simulink model "DC_Motor_speed_current_ctrl"  (R2021b)
settings: Solver=FixedStepAuto  StartTime=0.0  StopTime=2  FixedStep=5e-6  RelTol=1e-3
values from neighbouring files (symbols this model uses):
  B = 6.03e-6    (= 6.03e-06)    [DCMachine_cal.m]    (also in DC_Motor_speed_current_ctrl_cal.m = 0)
  I_rated = 74    [DC_Motor_speed_current_ctrl_cal.m]
  J = 1.06e-6    (= 1.06e-06)    [DCMachine_cal.m]    (also in DC_Motor_speed_current_ctrl_cal.m = 0.156)
  Kc = La/Td    (= 2.93)    [DC_Motor_speed_current_ctrl_cal.m]
  Kn = (J*K2)/(K1*Kphi*2*delta)    (= 65.9693860709)    [DC_Motor_speed_current_ctrl_cal.m]
  Kphi = 1.41e-2    (= 0.0141)    [DCMachine_cal.m]    (also in DC_Motor_speed_current_ctrl_cal.m = 1.18236661951)
  La = 120e-3    (= 0.12)    [DCMachine_cal.m]    (also in DC_Motor_speed_current_ctrl_cal.m = 0.00293)
  m_L = 0    [DC_Motor_speed_current_ctrl_cal.m]
  Ra = 7    [DCMachine_cal.m]    (also in DC_Motor_speed_current_ctrl_cal.m = 0.18)
  Tc = Ta    (= 0.0162777777778)    [DC_Motor_speed_current_ctrl_cal.m]
  Tn = 4*delta    (= 0.004)    [DC_Motor_speed_current_ctrl_cal.m]
  Vt = 6    [DCMachine_cal.m]    (also in DC_Motor_speed_current_ctrl_cal.m = 230)
  w_rpm = 1750    [DC_Motor_speed_current_ctrl_cal.m]
settings Model: Creator=jmvir  LastModifiedBy=Dinh-Tuyen Le

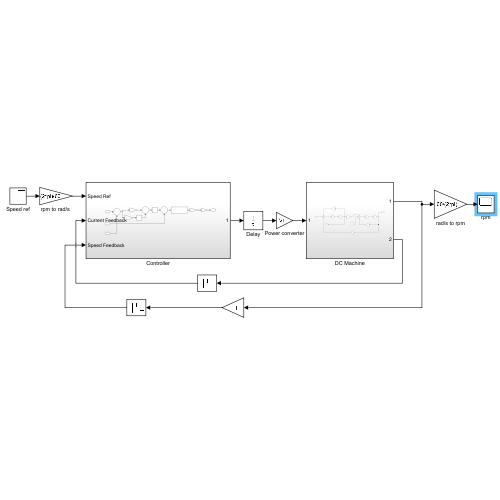
[thumbnail: Simulink's stored preview of the top-level diagram]
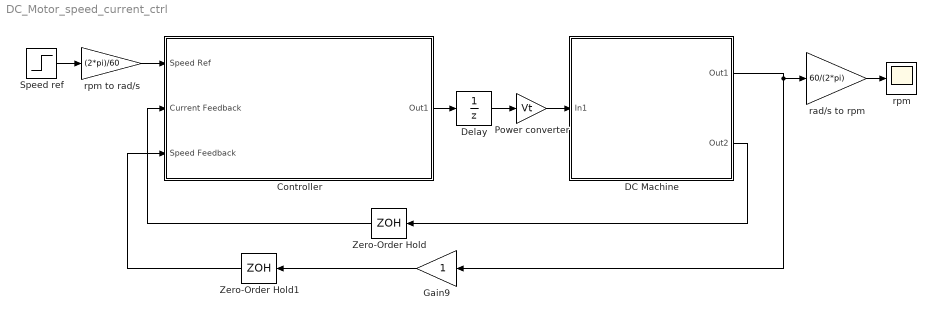
== system DC_Motor_speed_current_ctrl ==
  Controller : Subsystem
  DC Machine : Subsystem
  Delay : UnitDelay  SampleTime=-1  HasFrameUpgradeWarning=on
  Gain9 : Gain
  Power converter : Gain  Gain=Vt
  Speed ref : Step  Time=0  After=w_rpm  SampleTime=0
  Zero-Order Hold : ZeroOrderHold  SampleTime=-1
  Zero-Order Hold1 : ZeroOrderHold  SampleTime=-1
  rad/s to rpm : Gain  Gain=60/(2*pi)
  rpm : Scope
  "rpm to rad/s " : Gain  Gain=(2*pi)/60
  wires:
  Zero-Order Hold/1 -> Controller/2(Current Feedback)
  Gain9/1 -> Zero-Order Hold1/1
  Power converter/1 -> DC Machine/1(In1)
  Delay/1 -> Power converter/1
  Zero-Order Hold1/1 -> Controller/3(Speed Feedback)
  DC Machine/1(Out1) -> rad/s to rpm/1, Gain9/1
  Controller/1(Out1) -> Delay/1
  DC Machine/2(Out2) -> Zero-Order Hold/1
  rad/s to rpm/1 -> rpm/1
  "rpm to rad/s "/1 -> Controller/1(Speed Ref)
  Speed ref/1 -> "rpm to rad/s "/1

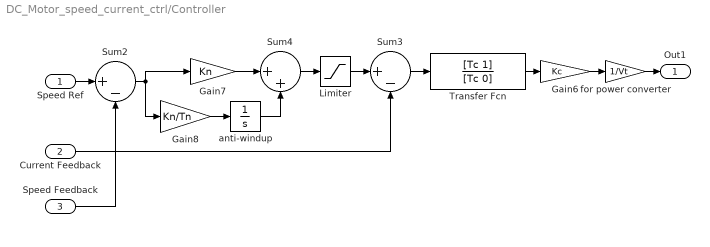
== system DC_Motor_speed_current_ctrl/Controller ==
  Speed Ref : Inport
  Current Feedback : Inport  Port=2
  Speed Feedback : Inport  Port=3
  Gain6 : Gain  Gain=Kc
  Gain7 : Gain  Gain=Kn
  Gain8 : Gain  Gain=Kn/Tn
  Limiter : Saturate  UpperLimit=I_rated  LowerLimit=-I_rated
  Sum2 : Sum  Inputs=|+-
  Sum3 : Sum  Inputs=|+-
  Sum4 : Sum  Inputs=|++
  Transfer Fcn : TransferFcn  Numerator=[Tc 1]  Denominator=[Tc 0]
  anti-windup : Integrator  LimitOutput=on  UpperSaturationLimit=I_rated  LowerSaturationLimit=-I_rated
  for power converter : Gain  Gain=1/Vt
  Out1 : Outport
  wires:
  Sum4/1 -> Limiter/1
  Sum3/1 -> Transfer Fcn/1
  Gain7/1 -> Sum4/1
  Sum2/1 -> Gain7/1, Gain8/1
  Limiter/1 -> Sum3/1
  Gain8/1 -> anti-windup/1
  Transfer Fcn/1 -> Gain6/1
  anti-windup/1 -> Sum4/2
  Speed Ref/1 -> Sum2/1
  Speed Feedback/1 -> Sum2/2
  Current Feedback/1 -> Sum3/2
  Gain6/1 -> for power converter/1
  for power converter/1 -> Out1/1

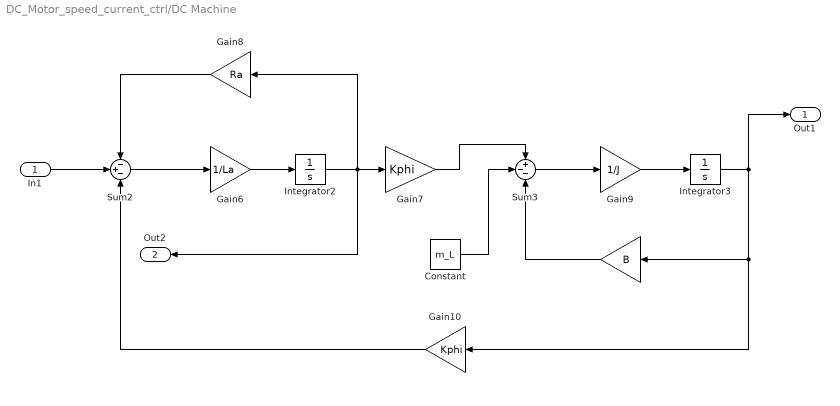
== system DC_Motor_speed_current_ctrl/DC Machine ==
  In1 : Inport
  " " : Gain  Gain=B
  Constant : Constant  Value=m_L
  Gain10 : Gain  Gain=Kphi
  Gain6 : Gain  Gain=1/La
  Gain7 : Gain  Gain=Kphi
  Gain8 : Gain  Gain=Ra
  Gain9 : Gain  Gain=1/J
  Integrator2 : Integrator
  Integrator3 : Integrator
  Sum2 : Sum  Inputs=-+-
  Sum3 : Sum  Inputs=+--
  Out1 : Outport
  Out2 : Outport  Port=2
  wires:
  Integrator2/1 -> Out2/1, Gain8/1, Gain7/1
  Constant/1 -> Sum3/2
  Gain9/1 -> Integrator3/1
  Gain10/1 -> Sum2/3
  " "/1 -> Sum3/3
  Sum3/1 -> Gain9/1
  Gain8/1 -> Sum2/1
  In1/1 -> Sum2/2
  Sum2/1 -> Gain6/1
  Integrator3/1 -> Out1/1, Gain10/1, " "/1
  Gain6/1 -> Integrator2/1
  Gain7/1 -> Sum3/1
